simulink model "AMCLIB_FWSpeedLoop_BAM"  (Simulink 9.3)
settings: Solver=VariableStepAuto  StartTime=0.0  StopTime=10.0  RelTol=1e-3
(part 2 of 2)

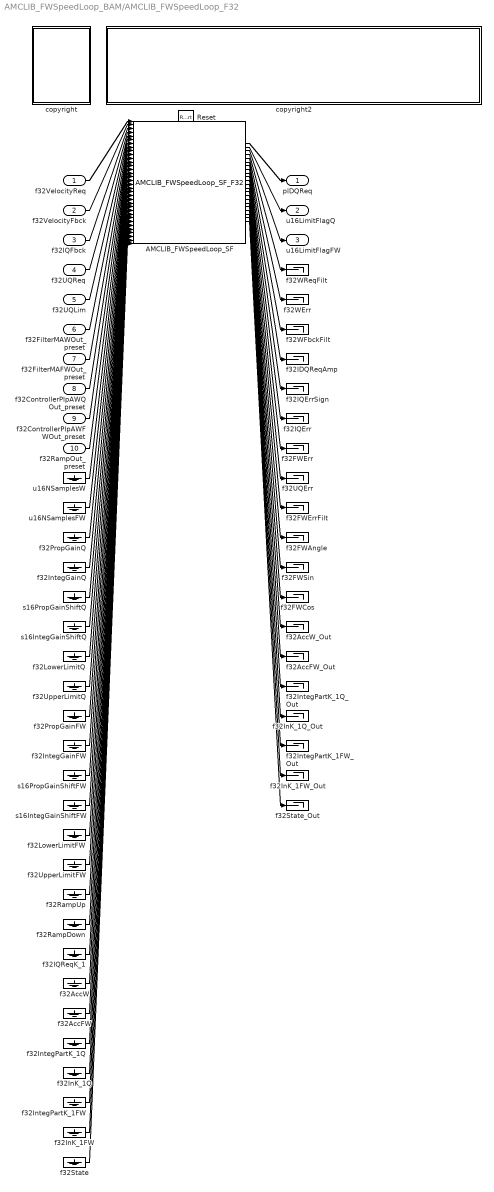
== system AMCLIB_FWSpeedLoop_BAM/AMCLIB_FWSpeedLoop_F32 ==
  f32VelocityReq : Inport  OutDataTypeStr=int32
  f32VelocityFbck : Inport  Port=2  OutDataTypeStr=int32
  f32IQFbck : Inport  Port=3  OutDataTypeStr=int32
  f32UQReq : Inport  Port=4  OutDataTypeStr=int32
  f32UQLim : Inport  Port=5  OutDataTypeStr=int32
  f32FilterMAWOut_preset : Inport  Port=6  OutDataTypeStr=int32
  f32FilterMAFWOut_preset : Inport  Port=7  OutDataTypeStr=int32
  f32ControllerPIpAWQOut_preset : Inport  Port=8  OutDataTypeStr=int32
  f32ControllerPIpAWFWOut_preset : Inport  Port=9  OutDataTypeStr=int32
  f32RampOut_preset : Inport  Port=10  OutDataTypeStr=int32
  Reset : ResetPort  DisableCoverage=on
  AMCLIB_FWSpeedLoop_SF : S-Function  FunctionName=AMCLIB_FWSpeedLoop_SF_F32  Parameters=showStates,resetStatesEnable,showDebugOutputs,u16NSamplesW,u16NSamplesFW,f32PropGainQ,f32IntegGainQ,s16PropGainShiftQ,s16IntegGainShiftQ,f32LowerLimitQ,f32UpperLimitQ,f32PropGainFW,f32IntegGainFW,s16PropGainShiftFW,s16IntegGainShiftFW,f32LowerLimitFW,f32UpperLimitFW,f32RampUp,f32RampDown  SFunctionDeploymentMode=off  EnableBusSupport=off
  copyright : Subsystem
      mask Display: text(10,90,'FILE:');text(10,75,'DESRIPTION:');text(10,60,'COPYRIGHT:');text(10,45,'VERSION:');text(10,30,'DATE:')
  copyright2 : Subsystem
      mask Display: text(10,90,'AMCLIB_FWSpeedLoop_BAM_F32.mdl');text(10,75,'PMSM Speed Loop with Field Weakening.');text(10,60,'NXP 2020');text(10,45,'1.0');text(10,30,'28-Mar-2020');
  f32AccFW : Ground
  f32AccFW_Out : Terminator
  f32AccW : Ground
  f32AccW_Out : Terminator
  f32FWAngle : Terminator
  f32FWCos : Terminator
  f32FWErr : Terminator
  f32FWErrFilt : Terminator
  f32FWSin : Terminator
  f32IDQReqAmp : Terminator
  f32IQErr : Terminator
  f32IQErrSign : Terminator
  f32IQReqK_1 : Ground
  f32InK_1FW : Ground
  f32InK_1FW_Out : Terminator
  f32InK_1Q : Ground
  f32InK_1Q_Out : Terminator
  f32IntegGainFW : Ground
  f32IntegGainQ : Ground
  f32IntegPartK_1FW : Ground
  f32IntegPartK_1FW_Out : Terminator
  f32IntegPartK_1Q : Ground
  f32IntegPartK_1Q_Out : Terminator
  f32LowerLimitFW : Ground
  f32LowerLimitQ : Ground
  f32PropGainFW : Ground
  f32PropGainQ : Ground
  f32RampDown : Ground
  f32RampUp : Ground
  f32State : Ground
  f32State_Out : Terminator
  f32UQErr : Terminator
  f32UpperLimitFW : Ground
  f32UpperLimitQ : Ground
  f32WErr : Terminator
  f32WFbckFilt : Terminator
  f32WReqFilt : Terminator
  s16IntegGainShiftFW : Ground
  s16IntegGainShiftQ : Ground
  s16PropGainShiftFW : Ground
  s16PropGainShiftQ : Ground
  u16NSamplesFW : Ground
  u16NSamplesW : Ground
  pIDQReq : Outport
  u16LimitFlagQ : Outport  Port=2
  u16LimitFlagFW : Outport  Port=3
  wires:
  f32VelocityReq/1 -> AMCLIB_FWSpeedLoop_SF/1
  f32VelocityFbck/1 -> AMCLIB_FWSpeedLoop_SF/2
  f32IQFbck/1 -> AMCLIB_FWSpeedLoop_SF/3
  f32UQReq/1 -> AMCLIB_FWSpeedLoop_SF/4
  f32UQLim/1 -> AMCLIB_FWSpeedLoop_SF/5
  f32FilterMAWOut_preset/1 -> AMCLIB_FWSpeedLoop_SF/6
  f32FilterMAFWOut_preset/1 -> AMCLIB_FWSpeedLoop_SF/7
  f32ControllerPIpAWQOut_preset/1 -> AMCLIB_FWSpeedLoop_SF/8
  f32ControllerPIpAWFWOut_preset/1 -> AMCLIB_FWSpeedLoop_SF/9
  f32RampOut_preset/1 -> AMCLIB_FWSpeedLoop_SF/10
  u16NSamplesW/1 -> AMCLIB_FWSpeedLoop_SF/11
  u16NSamplesFW/1 -> AMCLIB_FWSpeedLoop_SF/12
  f32PropGainQ/1 -> AMCLIB_FWSpeedLoop_SF/13
  f32IntegGainQ/1 -> AMCLIB_FWSpeedLoop_SF/14
  s16PropGainShiftQ/1 -> AMCLIB_FWSpeedLoop_SF/15
  s16IntegGainShiftQ/1 -> AMCLIB_FWSpeedLoop_SF/16
  f32LowerLimitQ/1 -> AMCLIB_FWSpeedLoop_SF/17
  f32UpperLimitQ/1 -> AMCLIB_FWSpeedLoop_SF/18
  f32PropGainFW/1 -> AMCLIB_FWSpeedLoop_SF/19
  f32IntegGainFW/1 -> AMCLIB_FWSpeedLoop_SF/20
  s16PropGainShiftFW/1 -> AMCLIB_FWSpeedLoop_SF/21
  s16IntegGainShiftFW/1 -> AMCLIB_FWSpeedLoop_SF/22
  f32LowerLimitFW/1 -> AMCLIB_FWSpeedLoop_SF/23
  f32UpperLimitFW/1 -> AMCLIB_FWSpeedLoop_SF/24
  f32RampUp/1 -> AMCLIB_FWSpeedLoop_SF/25
  f32RampDown/1 -> AMCLIB_FWSpeedLoop_SF/26
  f32IQReqK_1/1 -> AMCLIB_FWSpeedLoop_SF/27
  f32AccW/1 -> AMCLIB_FWSpeedLoop_SF/28
  f32AccFW/1 -> AMCLIB_FWSpeedLoop_SF/29
  f32IntegPartK_1Q/1 -> AMCLIB_FWSpeedLoop_SF/30
  f32InK_1Q/1 -> AMCLIB_FWSpeedLoop_SF/31
  f32IntegPartK_1FW/1 -> AMCLIB_FWSpeedLoop_SF/32
  f32InK_1FW/1 -> AMCLIB_FWSpeedLoop_SF/33
  f32State/1 -> AMCLIB_FWSpeedLoop_SF/34
  AMCLIB_FWSpeedLoop_SF/1 -> pIDQReq/1
  AMCLIB_FWSpeedLoop_SF/2 -> u16LimitFlagQ/1
  AMCLIB_FWSpeedLoop_SF/3 -> u16LimitFlagFW/1
  AMCLIB_FWSpeedLoop_SF/4 -> f32WReqFilt/1
  AMCLIB_FWSpeedLoop_SF/5 -> f32WErr/1
  AMCLIB_FWSpeedLoop_SF/6 -> f32WFbckFilt/1
  AMCLIB_FWSpeedLoop_SF/7 -> f32IDQReqAmp/1
  AMCLIB_FWSpeedLoop_SF/8 -> f32IQErrSign/1
  AMCLIB_FWSpeedLoop_SF/9 -> f32IQErr/1
  AMCLIB_FWSpeedLoop_SF/10 -> f32FWErr/1
  AMCLIB_FWSpeedLoop_SF/11 -> f32UQErr/1
  AMCLIB_FWSpeedLoop_SF/12 -> f32FWErrFilt/1
  AMCLIB_FWSpeedLoop_SF/13 -> f32FWAngle/1
  AMCLIB_FWSpeedLoop_SF/14 -> f32FWSin/1
  AMCLIB_FWSpeedLoop_SF/15 -> f32FWCos/1
  AMCLIB_FWSpeedLoop_SF/16 -> f32AccW_Out/1
  AMCLIB_FWSpeedLoop_SF/17 -> f32AccFW_Out/1
  AMCLIB_FWSpeedLoop_SF/18 -> f32IntegPartK_1Q_Out/1
  AMCLIB_FWSpeedLoop_SF/19 -> f32InK_1Q_Out/1
  AMCLIB_FWSpeedLoop_SF/20 -> f32IntegPartK_1FW_Out/1
  AMCLIB_FWSpeedLoop_SF/21 -> f32InK_1FW_Out/1
  AMCLIB_FWSpeedLoop_SF/22 -> f32State_Out/1

== system AMCLIB_FWSpeedLoop_BAM/AMCLIB_FWSpeedLoop_F32/copyright ==

== system AMCLIB_FWSpeedLoop_BAM/AMCLIB_FWSpeedLoop_F32/copyright2 ==
